simulink model "DD"  (R2021a)
settings: Solver=VariableStepAuto  StartTime=0.0  StopTime=10  RelTol=1e-3
undefined symbols (not defined in the file): B, K, M
settings Model: Creator=jaewan  LastModifiedBy=jaewan

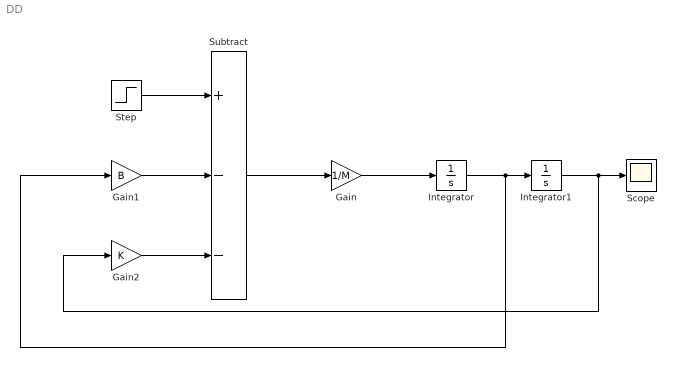
== system DD ==
  Gain : Gain  Gain=1/M
  Gain1 : Gain  Gain=B
  Gain2 : Gain  Gain=K
  Integrator : Integrator
  Integrator1 : Integrator
  Scope : Scope
  Step : Step  After=8  SampleTime=0
  Subtract : Sum  Inputs=+--
  wires:
  Subtract/1 -> Gain/1
  Integrator/1 -> Gain1/1, Integrator1/1
  Gain/1 -> Integrator/1
  Integrator1/1 -> Gain2/1, Scope/1
  Gain1/1 -> Subtract/2
  Gain2/1 -> Subtract/3
  Step/1 -> Subtract/1
